simulink model "BDamperError"  (R2024b)
settings: configuration reference "STM32H7_Config" (kept outside this file)
undefined symbols (not defined in the file): VDamperErrorHigh, VDamperErrorLow
libraries: simulink x8
settings Model: DataDictionary=Master_Dictionary.sldd  EnableAccessToBaseWorkspace=off  Creator=torni  LastModifiedBy=William
settings ConfigSetRef: SourceName=STM32H7_Config

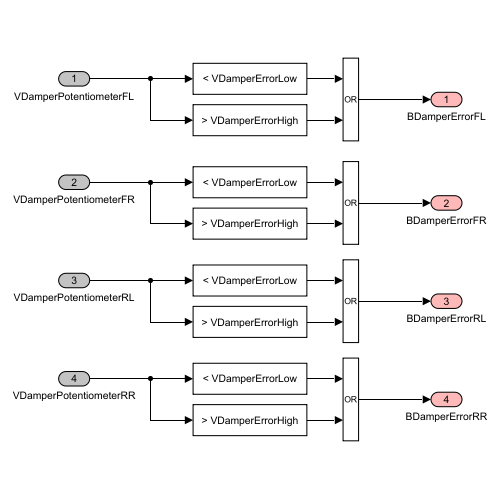
[thumbnail: Simulink's stored preview of the top-level diagram]
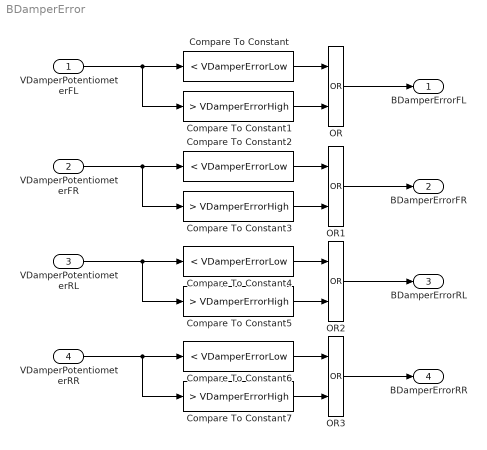
== system BDamperError ==
  VDamperPotentiometerFL : Inport  OutDataTypeStr=double
  "VDamperPotentiometerFR " : Inport  Port=2  OutDataTypeStr=double
  VDamperPotentiometerRL : Inport  Port=3  OutDataTypeStr=double
  VDamperPotentiometerRR : Inport  Port=4  OutDataTypeStr=double
  Compare To Constant{,2,4,6} (4 alike) : simulink/Logic and Bit Operations/Compare To Constant  relop=<  const=VDamperErrorLow  OutDataTypeStr=boolean
  Compare To Constant{1,3,5,7} (4 alike) : simulink/Logic and Bit Operations/Compare To Constant  relop=>  const=VDamperErrorHigh  OutDataTypeStr=boolean
  OR{,1..3} (4 alike) : Logic  Operator=OR  AllPortsSameDT=off  OutDataTypeStr=boolean
  BDamperErrorFL : Outport  OutDataTypeStr=boolean  VectorParamsAs1DForOutWhenUnconnected=off
  BDamperErrorFR : Outport  Port=2  OutDataTypeStr=boolean  VectorParamsAs1DForOutWhenUnconnected=off
  BDamperErrorRL : Outport  Port=3  OutDataTypeStr=boolean  VectorParamsAs1DForOutWhenUnconnected=off
  BDamperErrorRR : Outport  Port=4  OutDataTypeStr=boolean  VectorParamsAs1DForOutWhenUnconnected=off
  wires:
  Compare To Constant1/1 -> OR/2
  Compare To Constant/1 -> OR/1
  OR3/1 -> BDamperErrorRR/1
  VDamperPotentiometerFL/1 -> Compare To Constant1/1, Compare To Constant/1
  OR/1 -> BDamperErrorFL/1
  OR1/1 -> BDamperErrorFR/1
  "VDamperPotentiometerFR "/1 -> Compare To Constant2/1, Compare To Constant3/1
  Compare To Constant2/1 -> OR1/1
  Compare To Constant3/1 -> OR1/2
  Compare To Constant5/1 -> OR2/2
  Compare To Constant4/1 -> OR2/1
  VDamperPotentiometerRL/1 -> Compare To Constant5/1, Compare To Constant4/1
  OR2/1 -> BDamperErrorRL/1
  VDamperPotentiometerRR/1 -> Compare To Constant6/1, Compare To Constant7/1
  Compare To Constant6/1 -> OR3/1
  Compare To Constant7/1 -> OR3/2
